simulink library "INP_IMU_Comp2"  (R2023b)
settings: Solver=VariableStepAuto  StartTime=0.0  StopTime=10.0  RelTol=1e-3
undefined symbols (not defined in the file): INP_c_TiSample_s, INP_IMU_p_XPosImu_m, INP_IMU_p_YPosImu_m, INP_IMU_p_ZPosImu_m, INP_p_TiTau_s
libraries: matrix_library x3, VUT_lib x1
settings Model: Creator=blatak  LastModifiedBy=blatak

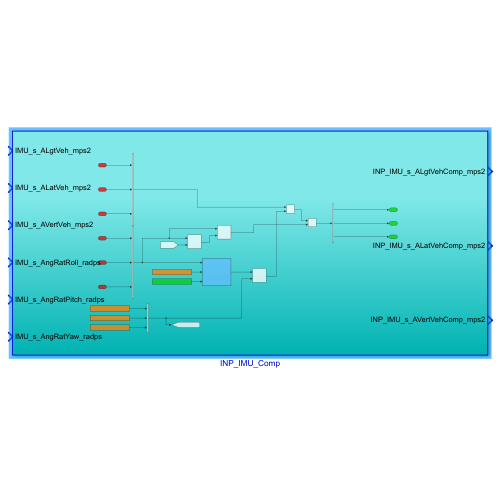
[thumbnail: Simulink's stored preview of the top-level diagram]
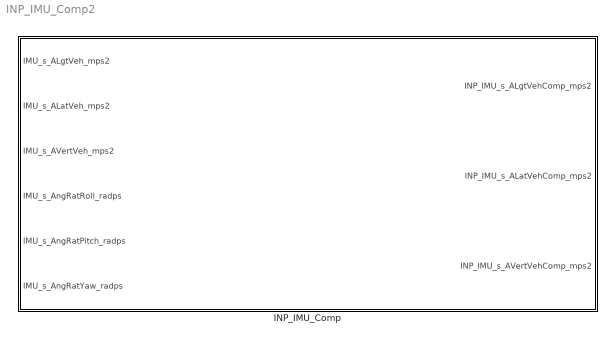
== system INP_IMU_Comp2 ==
  INP_IMU_Comp : Subsystem  Description=Block compensates measured accelerations from IMU position to cog

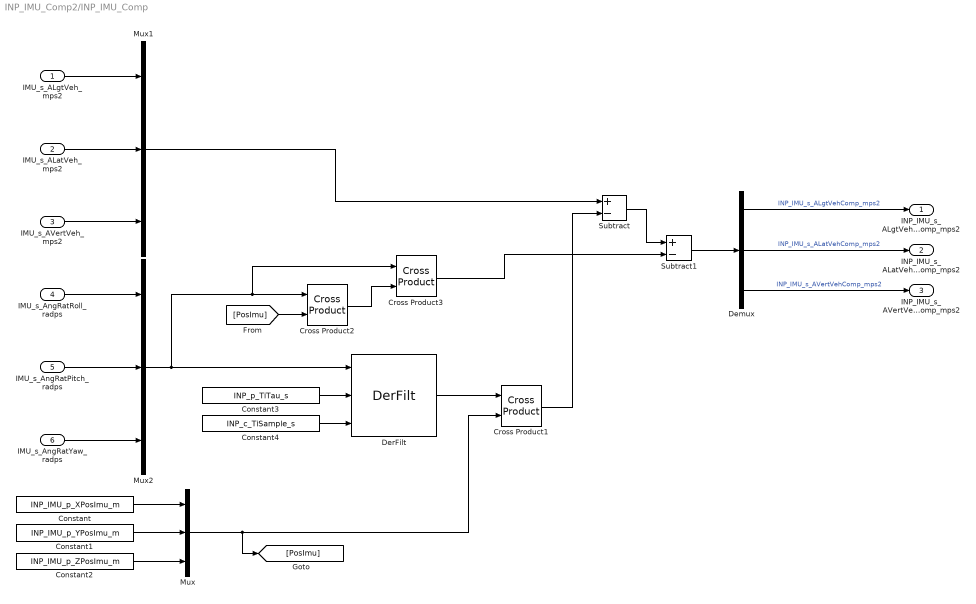
== system INP_IMU_Comp2/INP_IMU_Comp ==
  IMU_s_ALgtVeh_mps2 : Inport  Description=IMU Longitudinal acceleration - raw measured value from sensor
  IMU_s_ALatVeh_mps2 : Inport  Description=IMU Lateral acceleration - raw measured value from sensor  Port=2
  IMU_s_AVertVeh_mps2 : Inport  Description=IMU Vertical acceleration - raw measured value from sensor  Port=3
  IMU_s_AngRatRoll_radps : Inport  Description=IMU Angular roll velocity - raw measured value from sensor  Port=4
  IMU_s_AngRatPitch_radps : Inport  Description=IMU Angular pitch velocity - raw measured value from sensor  Port=5
  IMU_s_AngRatYaw_radps : Inport  Description=IMU Angular yaw velocity - raw measured value from sensor  Port=6
  Constant : Constant  Description=Position of the IMU to cog in x axis (longitudinal direction)  Value=INP_IMU_p_XPosImu_m
  Constant1 : Constant  Description=Position of the IMU to cog in y axis (lateral direction)  Value=INP_IMU_p_YPosImu_m
  Constant2 : Constant  Description=Position of the IMU to cog in z axis (vertical direction)  Value=INP_IMU_p_ZPosImu_m
  Constant3 : Constant  Value=INP_p_TiTau_s
  Constant4 : Constant  Description=Low pass filter block sampling time  Value=INP_c_TiSample_s
  Cross Product1 : matrix_library/Cross Product
  Cross Product2 : matrix_library/Cross Product
  Cross Product3 : matrix_library/Cross Product
  Demux : Demux  Outputs=3
  DerFilt : VUT_lib/DerFilt  SystemSampleTime=-1  VariantActivationTime=update diagram  AllowFlexibleInterface=on  Latency=0  AutoFrameSizeCalculation=off
  Mux : Mux  Inputs=3
  Mux1 : Mux  Inputs=3
  Mux2 : Mux  Inputs=3
  Subtract : Sum  Inputs=+-
  Subtract1 : Sum  Inputs=+-
  INP_IMU_s_ALgtVehComp_mps2 : Outport  Description=IMU Comp Longitudinal acceleration - compensated value - from IMU position to cog
  INP_IMU_s_ALatVehComp_mps2 : Outport  Description=IMU Comp Lateral acceleration - compensated value - from IMU position to cog  Port=2
  INP_IMU_s_AVertVehComp_mps2 : Outport  Description=IMU Comp Vertical acceleration - compensated value - from IMU position to cog  Port=3
  wires:
  Constant4/1 -> DerFilt/3
  Mux2/1 -> Cross Product3/1, Cross Product2/1, DerFilt/1
  Mux/1 -> [PosImu], Cross Product1/2
  DerFilt/1 -> Cross Product1/1
  Subtract1/1 -> Demux/1
  IMU_s_ALatVeh_mps2/1 -> Mux1/2
  Demux/1 -> INP_IMU_s_ALgtVehComp_mps2/1  "INP_IMU_s_ALgtVehComp_mps2"
  Cross Product1/1 -> Subtract/2
  IMU_s_AngRatYaw_radps/1 -> Mux2/3
  Constant3/1 -> DerFilt/2
  Constant2/1 -> Mux/3
  Subtract/1 -> Subtract1/1
  IMU_s_AVertVeh_mps2/1 -> Mux1/3
  Cross Product3/1 -> Subtract1/2
  Demux/2 -> INP_IMU_s_ALatVehComp_mps2/1  "INP_IMU_s_ALatVehComp_mps2"
  IMU_s_ALgtVeh_mps2/1 -> Mux1/1
  [PosImu] -> Cross Product2/2
  IMU_s_AngRatPitch_radps/1 -> Mux2/2
  Constant1/1 -> Mux/2
  Demux/3 -> INP_IMU_s_AVertVehComp_mps2/1  "INP_IMU_s_AVertVehComp_mps2"
  Mux1/1 -> Subtract/1
  Cross Product2/1 -> Cross Product3/2
  IMU_s_AngRatRoll_radps/1 -> Mux2/1
  Constant/1 -> Mux/1
